simulink model "LQR_simulink"  (R2021a)
settings: Solver=VariableStepAuto  StartTime=0.0  StopTime=200  RelTol=1e-3
values from neighbouring files (symbols this model uses):
  A = [0 1 0 0 0 0 0 0 0 0 0 0 ... (first row only)    [LQR_Weights_and_parameters.m]
  B = [0 0 0 0 0 0 ... (first row only)    [LQR_Weights_and_parameters.m]
  C = [1 0 0 0 0 0 0 0 0 0 0 0 ... (first row only)    [LQR_Weights_and_parameters.m]
  D = [0 0 0 0 0 0 ... (first row only)    [LQR_Weights_and_parameters.m]
  K = lqr(A,B,Q,R)    [LQR_Weights_and_parameters.m]
settings Model: Creator=zeray  LastModifiedBy=YEM
settings SolverCC: AlgebraicLoopSolver=TrustRegion
settings DataIOCC: SaveOutput=off  SaveTime=off  ReturnWorkspaceOutputs=off
settings DebuggingCC: SFMachineParentedDataDiag=warning

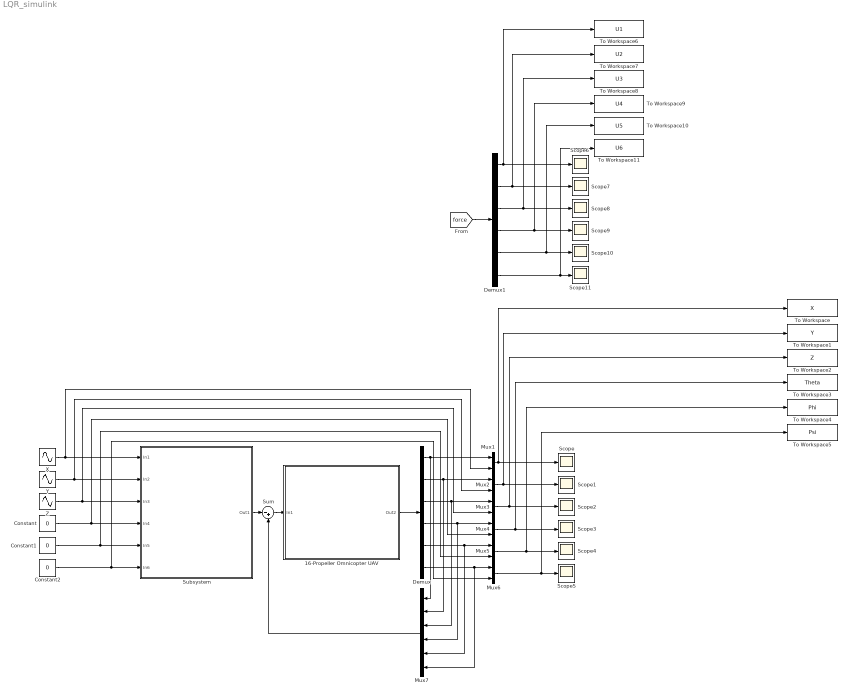
== system LQR_simulink ==
  16-Propeller Omnicopter UAV : Subsystem
      mask Display: image('$imagefile'); % Use "Edit Image" on toolstrip to change.
  Constant : Constant  Value=0
  Constant1 : Constant  Value=0
  Constant2 : Constant  Value=0
  Demux : Demux  Outputs=6
  Demux1 : Demux  Outputs=6
  Mux{1..6} (6 alike) : Mux  Inputs=2
  Mux7 : Mux  Inputs=6
  Scope{,1..11} (12 alike) : Scope
  Subsystem : Subsystem
  Sum : Sum  Inputs=|-+
  To Workspace : ToWorkspace  VariableName=X  SaveFormat=Timeseries  SampleTime=-1
  To Workspace1 : ToWorkspace  VariableName=Y  SaveFormat=Timeseries  SampleTime=-1
  To Workspace10 : ToWorkspace  VariableName=U5  SaveFormat=Timeseries  SampleTime=-1
  To Workspace11 : ToWorkspace  VariableName=U6  SaveFormat=Timeseries  SampleTime=-1
  To Workspace2 : ToWorkspace  VariableName=Z  SaveFormat=Timeseries  SampleTime=-1
  To Workspace3 : ToWorkspace  VariableName=Theta  SaveFormat=Timeseries  SampleTime=-1
  To Workspace4 : ToWorkspace  VariableName=Phi  SaveFormat=Timeseries  SampleTime=-1
  To Workspace5 : ToWorkspace  VariableName=Psi  SaveFormat=Timeseries  SampleTime=-1
  To Workspace6 : ToWorkspace  VariableName=U1  SaveFormat=Timeseries  SampleTime=-1
  To Workspace7 : ToWorkspace  VariableName=U2  SaveFormat=Timeseries  SampleTime=-1
  To Workspace8 : ToWorkspace  VariableName=U3  SaveFormat=Timeseries  SampleTime=-1
  To Workspace9 : ToWorkspace  VariableName=U4  SaveFormat=Timeseries  SampleTime=-1
  X : Sin  Amplitude=20  Frequency=0.1  Phase=1.57  SampleTime=0
  Y : Sin  Amplitude=20  Frequency=0.1  SampleTime=0
  Z : Sin  Amplitude=100  Frequency=0.04  SampleTime=0
  wires:
  X/1 -> Subsystem/1(In1), Mux1/2
  Z/1 -> Subsystem/3(In3), Mux3/2
  Y/1 -> Subsystem/2(In2), Mux2/2
  Mux1/1 -> To Workspace/1, Scope/1
  Mux2/1 -> To Workspace1/1, Scope1/1
  Mux3/1 -> To Workspace2/1, Scope2/1
  Mux4/1 -> Scope3/1, To Workspace3/1
  Mux5/1 -> Scope4/1, To Workspace4/1
  Mux6/1 -> Scope5/1, To Workspace5/1
  Demux/1 -> Mux7/1, Mux1/1
  Demux/2 -> Mux7/2, Mux2/1
  Demux/3 -> Mux7/3, Mux3/1
  Demux/4 -> Mux7/4, Mux4/1
  Demux/5 -> Mux7/5, Mux5/1
  Demux/6 -> Mux7/6, Mux6/1
  Demux1/1 -> Scope6/1, To Workspace6/1
  Demux1/2 -> To Workspace7/1, Scope7/1
  Demux1/3 -> Scope8/1, To Workspace8/1
  Demux1/4 -> Scope9/1, To Workspace9/1
  Demux1/5 -> Scope10/1, To Workspace10/1
  Demux1/6 -> Scope11/1, To Workspace11/1
  Mux7/1 -> Sum/2
  Constant/1 -> Subsystem/4(In4), Mux4/2
  Constant1/1 -> Mux5/2, Subsystem/5(In5)
  Constant2/1 -> Subsystem/6(In6), Mux6/2
  Subsystem/1(Out1) -> Sum/1
  Sum/1 -> 16-Propeller Omnicopter UAV/1(In1)
  16-Propeller Omnicopter UAV/1(Out2) -> Demux/1
  [force] -> Demux1/1

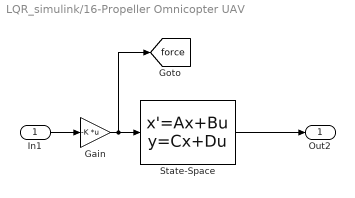
== system LQR_simulink/16-Propeller Omnicopter UAV ==
  In1 : Inport
  Gain : Gain  Gain=-K  Multiplication=Matrix(K*u)
  State-Space : StateSpace  A=A  B=B  C=C  D=D  InitialCondition=0
  Out2 : Outport
  tag scope: force=global
  wires:
  State-Space/1 -> Out2/1
  Gain/1 -> [force], State-Space/1
  In1/1 -> Gain/1

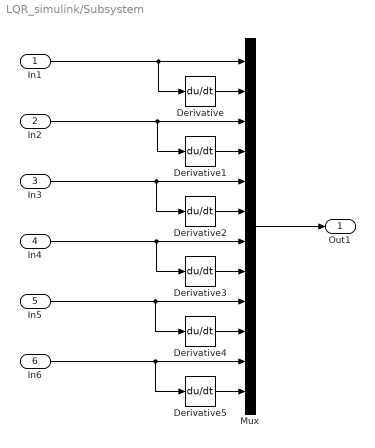
== system LQR_simulink/Subsystem ==
  In1 : Inport
  In2 : Inport  Port=2
  In3 : Inport  Port=3
  In4 : Inport  Port=4
  In5 : Inport  Port=5
  In6 : Inport  Port=6
  Derivative{,1..5} (6 alike) : Derivative
  Mux : Mux  Inputs=12
  Out1 : Outport
  wires:
  Derivative2/1 -> Mux/6
  In6/1 -> Derivative5/1, Mux/11
  In1/1 -> Derivative/1, Mux/1
  In2/1 -> Mux/3, Derivative1/1
  In4/1 -> Mux/7, Derivative3/1
  In3/1 -> Mux/5, Derivative2/1
  In5/1 -> Mux/9, Derivative4/1
  Derivative1/1 -> Mux/4
  Derivative5/1 -> Mux/12
  Derivative4/1 -> Mux/10
  Derivative3/1 -> Mux/8
  Derivative/1 -> Mux/2
  Mux/1 -> Out1/1
